simulink model "sf_eventfcn"  (Simulink 6.0)
settings: Solver=ode45  StartTime=0.0  StopTime=30  MaxStep=1  RelTol=1e-3
settings Model: CovMetricSettings=dcmtr  Creator=The MathWorks Inc.  LastModifiedBy=batserve  ExtModeAutoUpdateStatusClock=off
settings DataIOCC: SignalLoggingName=sigsOut
settings OptimizationCC: BooleanDataType=off
settings DebuggingCC: CheckExecutionContextPreStartOutputMsg=on  CheckExecutionContextRuntimeOutputMsg=on  SolverPrmCheckMsg=none
settings HardwareCC: TargetUnknown=on

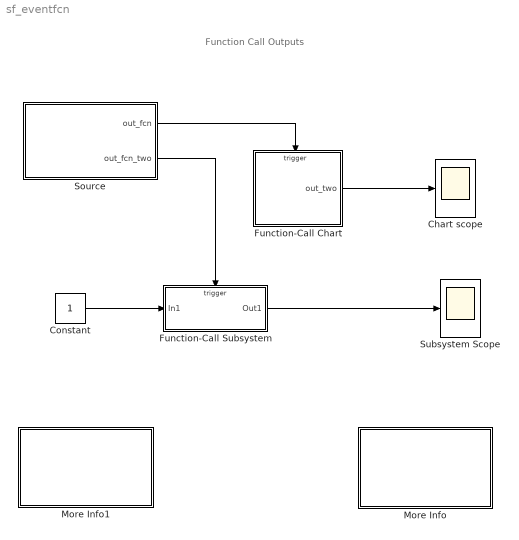
== system sf_eventfcn ==
  note: Function Call Outputs
  Chart scope : Scope
      settings: TimeRange=30  YMin=0  YMax=1
  Constant : Constant
  Function-Call Subsystem : Subsystem  TreatAsAtomicUnit=on  PropExecContextAcrossSSBoundary=on
  Function-Call Chart : Stateflow chart  TreatAsAtomicUnit=on  PropExecContextAcrossSSBoundary=on
  More Info : Subsystem  PropExecContextAcrossSSBoundary=on
      mask Display: disp('Double click\nhere for\ninformation on\nthis demonstration')
  More Info1 : Subsystem  PropExecContextAcrossSSBoundary=on
      settings: OpenFcn=simcad(bdroot);
      mask Display: disp('Double click\nhere for\nSimulink\Stateflow\n Help')
  Source : Stateflow chart  PropExecContextAcrossSSBoundary=on
  Subsystem Scope : Scope
      settings: TimeRange=30  YMin=0  YMax=2
  wires:
  Source/2(out_fcn_two) -> Function-Call Subsystem/Trigger
  Source/1(out_fcn) -> Function-Call Chart/Trigger
  Function-Call Chart/1(out_two) -> Chart scope/1
  Constant/1 -> Function-Call Subsystem/1(In1)
  Function-Call Subsystem/1(Out1) -> Subsystem Scope/1

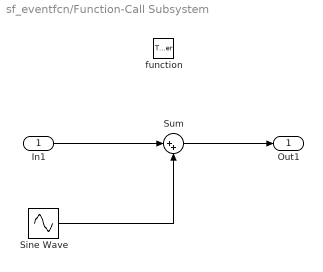
== system sf_eventfcn/Function-Call Subsystem ==
  In1 : Inport  Port=1  LatchInput=off
  function : TriggerPort  TriggerType=function-call  ZeroCross=off
  Sine Wave : Sin
  Sum : Sum  Inputs=|++  SaturateOnIntegerOverflow=on  InputSameDT=on
  Out1 : Outport
  wires:
  In1/1 -> Sum/1
  Sum/1 -> Out1/1
  Sine Wave/1 -> Sum/2

== system sf_eventfcn/More Info ==
  note: Function Call Outputs
  note: Function call outputs are used to control the activation times of other Stateflow charts or subsystems.
      | This demonstration illustrates how a control Stateflow chart, named 'Source', determines the activation
      | times of another Stateflow chart and also function-call subsystem. The 'Function-Call Chart' is activated
      | after every '3' simulation time steps by the function-call signal 'out_fcn'. The 'Function-call Subsystem'
      | is activated every 2 time steps by receiving the function call signal named 'out_fcn_two'.
      |
      | Notice that in the output plots, the time distance between each sample point is 3 for the
      | 'Function-Call Chart and 2 for the function-call subsystem. This is easier to view if you zoom into
      | the x-axis of the plots.

== system sf_eventfcn/More Info1 ==

== stateflow chart Source ==
  state One [parallel]
    state A
    A -> A : after(3,wakeup)/out_fcn;
  state Two [parallel]
    state B
    (default) -> B
    B -> B : after(2,wakeup)/out_fcn_two;
  (default) -> A
  data: local_count local double
  events: out_fcn output FUNCTION_CALL_EVENT; out_fcn_two output FUNCTION_CALL_EVENT

== stateflow chart Function-Call Chart ==
  state A
    en:out_two=0;
  state B
    en:out_two=1;
  (default) -> A
  A -> B
  B -> A
  data: out_two output double
  events: event input FUNCTION_CALL_EVENT
